simulink model "RL_circuit"  (R2024b)
settings: Solver=VariableStepAuto  StartTime=0.0  StopTime=5.0  RelTol=1e-3
undefined symbols (not defined in the file): denCi, denT, Kg, numCi, numT, R
libraries: simulink_extras x3
settings Model: Creator=edoardo  LastModifiedBy=edoardo

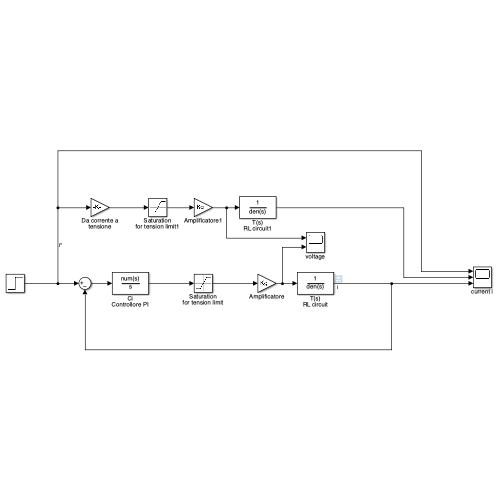
[thumbnail: Simulink's stored preview of the top-level diagram]
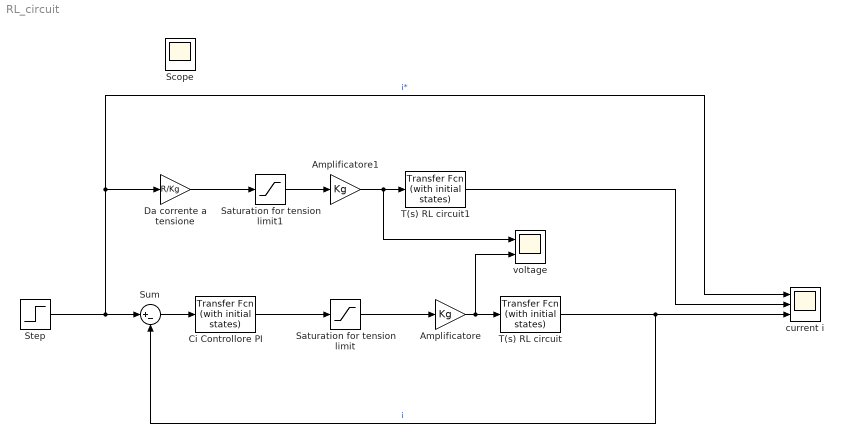
== system RL_circuit ==
  Amplificatore : Gain  Gain=Kg
  Amplificatore1 : Gain  Gain=Kg
  Ci Controllore PI : simulink_extras/Additional Linear/Transfer Fcn (with initial states)  N=numCi  D=denCi  X0=0
  Da corrente a tensione : Gain  Gain=R/Kg
  Saturation for tension limit : Saturate  UpperLimit=8  LowerLimit=-8
  Saturation for tension limit1 : Saturate  UpperLimit=8  LowerLimit=-8
  Step : Step  SampleTime=0
  Sum : Sum  Inputs=|+-
  T(s) RL circuit : simulink_extras/Additional Linear/Transfer Fcn (with initial states)  N=numT  D=denT  X0=0
  T(s) RL circuit1 : simulink_extras/Additional Linear/Transfer Fcn (with initial states)  N=numT  D=denT  X0=0
  current i : Scope  NumInputPorts=3
  voltage : Scope  NumInputPorts=2
  Scope : Scope
  wires:
  Amplificatore/1 -> voltage/2, T(s) RL circuit/1
  T(s) RL circuit/1 -> Sum/2, current i/3  "i"
  Sum/1 -> Ci Controllore PI/1
  Saturation for tension limit/1 -> Amplificatore/1
  Ci Controllore PI/1 -> Saturation for tension limit/1
  Step/1 -> Da corrente a tensione/1, current i/1, Sum/1  "i*"
  Amplificatore1/1 -> voltage/1, T(s) RL circuit1/1
  Saturation for tension limit1/1 -> Amplificatore1/1
  Da corrente a tensione/1 -> Saturation for tension limit1/1
  T(s) RL circuit1/1 -> current i/2
